simulink model "rangeSensorSoln"  (R2018a)
settings: Solver=FixedStepDiscrete  StartTime=0.0  StopTime=10.0  RelTol=1e-3  EnableMultiTasking=on
PreLoadFcn:
  | tFilter = 0.01;
  | tFusion = 0.05;
  | 
  | sensData = dlmread('rangeSensorData.txt');
settings Model: Creator=scastro  LastModifiedBy=scastro
settings DataIOCC: ExternalInput=sensData  LoadExternalInput=on
settings OptimizationCC: DefaultParameterBehavior=Inlined  EnhancedBackFolding=on  PassReuseOutputArgsAs=Individual arguments  OptimizeBlockOrder=speed  DifferentSizesBufferReuse=on  OptimizationCustomize=off
settings DebuggingCC: ParameterTunabilityLossMsg=error  LibraryContextMissingDiagnostic=warning
settings SFSimCC: SimUseLocalCustomCode=on  MATLABDynamicMemAlloc=off
settings RTWCC: SystemTargetFile=ert.tlc  TemplateMakefile=ert_default_tmf  GenerateReport=on  RTWUseLocalCustomCode=on  IncludeHyperlinkInReport=on  LaunchReport=on  GenerateTraceInfo=on  GenerateTraceReport=on  GenerateTraceReportSl=on  GenerateTraceReportSf=on  GenerateTraceReportEml=on
settings CodeAppCC: ForceParamTrailComments=on  IgnoreCustomStorageClasses=off  OperatorAnnotations=on  SimulinkDataObjDesc=on  SFDataObjDesc=on  InsertBlockDesc=on
settings ERTTargetCC: TargetLangStandard=C99 (ISO)  GenerateSampleERTMain=on  InlinedParameterPlacement=NonHierarchical  ERTCustomFileTemplate=example_file_process.tlc

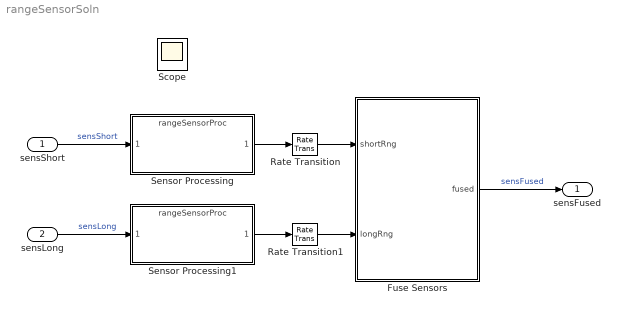
== system rangeSensorSoln ==
  sensShort : Inport
  sensLong : Inport  Port=2
  Fuse Sensors : Stateflow chart  TreatAsAtomicUnit=on  SystemSampleTime=tFusion
  Rate Transition : RateTransition
  Rate Transition1 : RateTransition
  Sensor Processing : ModelReference  ModelNameDialog=rangeSensorProc  SimulationMode=Normal  ModelReferenceVersion=1.9
  Sensor Processing1 : ModelReference  ModelNameDialog=rangeSensorProc  SimulationMode=Normal  ModelReferenceVersion=1.9
  sensFused : Outport
  Scope : Scope
  wires:
  Sensor Processing/1 -> Rate Transition/1
  sensShort/1 -> Sensor Processing/1  "sensShort"
  Sensor Processing1/1 -> Rate Transition1/1
  sensLong/1 -> Sensor Processing1/1  "sensLong"
  Fuse Sensors/1(fused) -> sensFused/1  "sensFused"
  Rate Transition/1 -> Fuse Sensors/1(shortRng)
  Rate Transition1/1 -> Fuse Sensors/2(longRng)

== stateflow chart rangeSensorSoln/Fuse Sensors ==
  state AverageReadings
    en,du:
    fused = 0.5*(shortRng + longRng);
  state ShortRange
    en,du:
    fused = shortRng;
  state LongRange
    en,du:
    fused = longRng;
  (default) -> AverageReadings
  AverageReadings -> LongRange [order 2] : [fused > 80]
  AverageReadings -> ShortRange [order 1] : [fused < 40]
  LongRange -> AverageReadings : [fused <= 80]
  ShortRange -> AverageReadings : [fused >= 40]
  data: shortRng input; longRng input; fused output
